simulink model "MPC_temp_arduino"  (R2021a)
settings: Solver=VariableStepAuto  StartTime=0.0  StopTime=10.0  RelTol=1e-3
values from neighbouring files (symbols this model uses):
  A = [0,                              1,                                                           0,                                                            0 ... (first row only)    [ss_mpc.m]    (also in tumbllerDT0.m = [3.9200 -5.7860 3.8100 -0.9451;1 0 0 0;0 1 0 0;0 0 1 0]; tumbller_mpc.m)
  B = v_to_force*[               0 ... (first row only)    [ss_mpc.m]    (also in tumbllerDT0.m = [1;0;0;0]; tumbller_mpc.m = [               0)
  f = 0.01    [ss_mpc.m]    (also in tumbller_mpc.m)
  g = 9.81    [ss_mpc.m]    (also in tumbller_mpc.m)
  I_pend = 0.00024    [ss_mpc.m]    (also in tumbller_mpc.m)
  l = 0.04    [ss_mpc.m]    (also in tumbller_mpc.m)
  m_cart = 0.493    [ss_mpc.m]    (also in tumbller_mpc.m)
  m_pend = 0.312    [ss_mpc.m]    (also in tumbller_mpc.m)
  v_to_force = (2*kT)/(R*r)    (= 0.65671641791)    [ss_mpc.m]    (also in tumbller_mpc.m)
libraries: pid_lib x2, mpclib x1, simulink x1
settings Model: Creator=navoditchandra  LastModifiedBy=navoditchandra

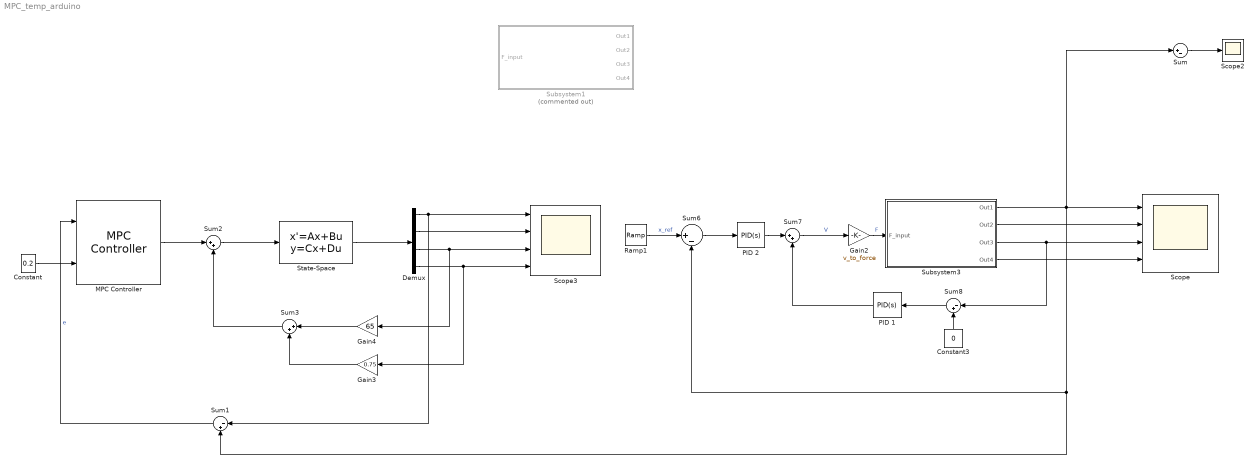
== system MPC_temp_arduino ==
  Constant : Constant  Value=0.2
  Constant3 : Constant  Value=0
  Demux : Demux
  Gain2 : Gain  Gain=v_to_force
  Gain3 : Gain  Gain=0.75
  Gain4 : Gain  Gain=65
  MPC Controller : mpclib/MPC Controller  SCDEnableBlockLinearizationSpecification=on  mpcobj=mpc1  is_multiple=0  enable_value=0  return_u0=off  updateMPCinCallerWorkspace=on  md_inport=off  mv_inport=off  uref_inport=off  return_cost=off  return_mvseq=off  return_qpstatus=off  return_xseq=off  return_state=off  return_ovseq=off  state_inport=off  umin_inport=off  umax_inport=off  ymin_inport=off  ymax_inport=off  cc_inport=off  ywt_inport=off  uwt_inport=off  duwt_inport=off  rhoeps_inport=off  pm_inport=off  MaximumP=10  HorizonChoice=FixedHorizon  n_ts=0.02  n_p=10  n_mv=1  n_md=0  n_ud=0  n_mo=1  n_uo=0  BlockDataType=double  SampleTimeInherited=off  switch_inport=off
  PID 1 : pid_lib/PID Controller  Controller=PID  Form=Parallel  TimeDomain=Continuous-time  UseExternalTs=off  SampleTime=-1  IntegratorMethod=Forward Euler  FilterMethod=Forward Euler  ControllerParametersSource=internal  P=-887.275388547678  I=-21478.8660944054  D=-9.12643726781358  UseFilter=on  N=21022.2428165113  TunerSelectOption=Transfer Function Based (PID Tuner App)  InitialConditionSource=internal  InitialConditionForIntegrator=0  InitialConditionForFilter=0  DifferentiatorICPrevScaledInput=0  ExternalReset=none  TrackingMode=off  Kt=1  LimitOutput=off  SatLimitsSource=internal  UpperSaturationLimit=inf  LowerSaturationLimit=-inf  LinearizeAsGain=on  AntiWindupMode=none  Kb=1  POutMin=[]  POutMax=[]  IOutMin=[]  IOutMax=[]  DOutMin=[]  DOutMax=[]  NOutMin=[]  NOutMax=[]  SumOutMin=[]  SumOutMax=[]  SaturationOutMin=[]  SaturationOutMax=[]  PParamMin=[]  PParamMax=[]  IParamMin=[]  IParamMax=[]  DParamMin=[]  DParamMax=[]  NParamMin=[]  NParamMax=[]  KbParamMin=[]  KbParamMax=[]  KtParamMin=[]  KtParamMax=[]  KbOutMin=[]  KbOutMax=[]  KtOutMin=[]  KtOutMax=[]  IntegratorOutMin=[]  IntegratorOutMax=[]  FilterOutMin=[]  FilterOutMax=[]  SumI1OutMin=[]  SumI1OutMax=[]  SumI2OutMin=[]  SumI2OutMax=[]  SumI3OutMin=[]  SumI3OutMax=[]  SumI4OutMin=[]  SumI4OutMax=[]  SumDOutMin=[]  SumDOutMax=[]  DifferentiatorOutMin=[]  DifferentiatorOutMax=[]  FilterDiffOutCoefMin=[]  FilterDiffOutCoefMax=[]  ReciprocalOutMin=[]  ReciprocalOutMax=[]  SumDenOutMin=[]  SumDenOutMax=[]  SumNumOutMin=[]  SumNumOutMax=[]  DivideOutMin=[]  DivideOutMax=[]  UdiffTsProdOutMin=[]  UdiffTsProdOutMax=[]  NTsProdOutMin=[]  NTsProdOutMax=[]  UintegralTsProdOutMin=[]  UintegralTsProdOutMax=[]  UngainTsProdOutMin=[]  UngainTsProdOutMax=[]  IntegratorContinuousStateAttributes=''  IntegratorStateMustResolveToSignalObject=off  IntegratorRTWStateStorageClass=Auto  FilterContinuousStateAttributes=''  FilterStateMustResolveToSignalObject=off  FilterRTWStateStorageClass=Auto  ParallelPVariant=InternalParameters  IdealPVariant=Disabled  IVariant=InternalParameters  DVariant=InternalParameters  IntegratorVariant=Continuous  SatVariant=Disabled  AWVariant=Passthrough  PCopyVariant=Disabled  TRVariant=Disabled  FdbkBlocksVariant=Forward  IdealPFdbkVariant=Disabled  SatFdbkVariant=Disabled  DerivativeFilterVariant=ContFilter  NVariant=InternalParameters  NCopyVariant=Disabled  FilterICVariant=InternalICsFilter  IntegratorICVariant=InternalICs  ExternalResetVariant=Disabled  TRSumVariant=Passthrough  SumFdbkVariant=Disabled  SumVariant=Sum_PID  TsampFilterVariant=InternalTs  TsampNgainVariant=Passthrough  TsampIntegralVariant=Passthrough  ExternalSaturationOutDataTypeStr=Inherit: Same as second input
  PID 2 : pid_lib/PID Controller  Controller=PID  Form=Parallel  TimeDomain=Continuous-time  UseExternalTs=off  SampleTime=-1  IntegratorMethod=Forward Euler  FilterMethod=Forward Euler  ControllerParametersSource=internal  P=19501.8727650453  I=12310.6101317188  D=-477.528521319051  UseFilter=on  N=35.5633957258041  TunerSelectOption=Transfer Function Based (PID Tuner App)  InitialConditionSource=internal  InitialConditionForIntegrator=0  InitialConditionForFilter=0  DifferentiatorICPrevScaledInput=0  ExternalReset=none  TrackingMode=off  Kt=1  LimitOutput=off  SatLimitsSource=internal  UpperSaturationLimit=inf  LowerSaturationLimit=-inf  LinearizeAsGain=on  AntiWindupMode=none  Kb=1  POutMin=[]  POutMax=[]  IOutMin=[]  IOutMax=[]  DOutMin=[]  DOutMax=[]  NOutMin=[]  NOutMax=[]  SumOutMin=[]  SumOutMax=[]  SaturationOutMin=[]  SaturationOutMax=[]  PParamMin=[]  PParamMax=[]  IParamMin=[]  IParamMax=[]  DParamMin=[]  DParamMax=[]  NParamMin=[]  NParamMax=[]  KbParamMin=[]  KbParamMax=[]  KtParamMin=[]  KtParamMax=[]  KbOutMin=[]  KbOutMax=[]  KtOutMin=[]  KtOutMax=[]  IntegratorOutMin=[]  IntegratorOutMax=[]  FilterOutMin=[]  FilterOutMax=[]  SumI1OutMin=[]  SumI1OutMax=[]  SumI2OutMin=[]  SumI2OutMax=[]  SumI3OutMin=[]  SumI3OutMax=[]  SumI4OutMin=[]  SumI4OutMax=[]  SumDOutMin=[]  SumDOutMax=[]  DifferentiatorOutMin=[]  DifferentiatorOutMax=[]  FilterDiffOutCoefMin=[]  FilterDiffOutCoefMax=[]  ReciprocalOutMin=[]  ReciprocalOutMax=[]  SumDenOutMin=[]  SumDenOutMax=[]  SumNumOutMin=[]  SumNumOutMax=[]  DivideOutMin=[]  DivideOutMax=[]  UdiffTsProdOutMin=[]  UdiffTsProdOutMax=[]  NTsProdOutMin=[]  NTsProdOutMax=[]  UintegralTsProdOutMin=[]  UintegralTsProdOutMax=[]  UngainTsProdOutMin=[]  UngainTsProdOutMax=[]  IntegratorContinuousStateAttributes=''  IntegratorStateMustResolveToSignalObject=off  IntegratorRTWStateStorageClass=Auto  FilterContinuousStateAttributes=''  FilterStateMustResolveToSignalObject=off  FilterRTWStateStorageClass=Auto  ParallelPVariant=InternalParameters  IdealPVariant=Disabled  IVariant=InternalParameters  DVariant=InternalParameters  IntegratorVariant=Continuous  SatVariant=Disabled  AWVariant=Passthrough  PCopyVariant=Disabled  TRVariant=Disabled  FdbkBlocksVariant=Forward  IdealPFdbkVariant=Disabled  SatFdbkVariant=Disabled  DerivativeFilterVariant=ContFilter  NVariant=InternalParameters  NCopyVariant=Disabled  FilterICVariant=InternalICsFilter  IntegratorICVariant=InternalICs  ExternalResetVariant=Disabled  TRSumVariant=Passthrough  SumFdbkVariant=Disabled  SumVariant=Sum_PID  TsampFilterVariant=InternalTs  TsampNgainVariant=Passthrough  TsampIntegralVariant=Passthrough  ExternalSaturationOutDataTypeStr=Inherit: Same as second input
  Ramp1 : simulink/Sources/Ramp  slope=1  start=0  InitialOutput=0
  Scope : Scope  NumInputPorts=4
  Scope2 : Scope
  Scope3 : Scope  NumInputPorts=4
  State-Space : StateSpace  A=A  B=B  C=eye(4)  D=zeros(4,1)  InitialCondition=-0.2
  Subsystem1 : Subsystem  Commented=on
  Subsystem3 : Subsystem
  Sum : Sum  Inputs=|+-
  Sum1 : Sum  Inputs=|-+
  Sum2 : Sum  Inputs=|++
  Sum3 : Sum  Inputs=|++
  Sum6 : Sum  Inputs=|+-
  Sum7 : Sum  Inputs=|++
  Sum8 : Sum  Inputs=|-+
  wires:
  Sum6/1 -> PID 2/1
  PID 1/1 -> Sum7/2
  Subsystem3/1(Out1) -> Sum/1, Sum1/2, Sum6/2, Scope/1
  Sum/1 -> Scope2/1
  MPC Controller/1 -> Sum2/1
  Sum7/1 -> Gain2/1  "V"
  Sum8/1 -> PID 1/1
  Sum2/1 -> State-Space/1
  Sum1/1 -> MPC Controller/1  "e"
  Constant/1 -> MPC Controller/2
  Subsystem3/2(Out2) -> Scope/2
  Gain2/1 -> Subsystem3/1(F_input)  "F"
  Subsystem3/4(Out4) -> Scope/4
  PID 2/1 -> Sum7/1
  Subsystem3/3(Out3) -> Sum8/1, Scope/3
  Ramp1/1 -> Sum6/1  "x_ref"
  Constant3/1 -> Sum8/2
  Gain4/1 -> Sum3/1
  Gain3/1 -> Sum3/2
  Sum3/1 -> Sum2/2
  State-Space/1 -> Demux/1
  Demux/3 -> Scope3/3, Gain4/1
  Demux/4 -> Scope3/4, Gain3/1
  Demux/1 -> Sum1/1, Scope3/1
  Demux/2 -> Scope3/2

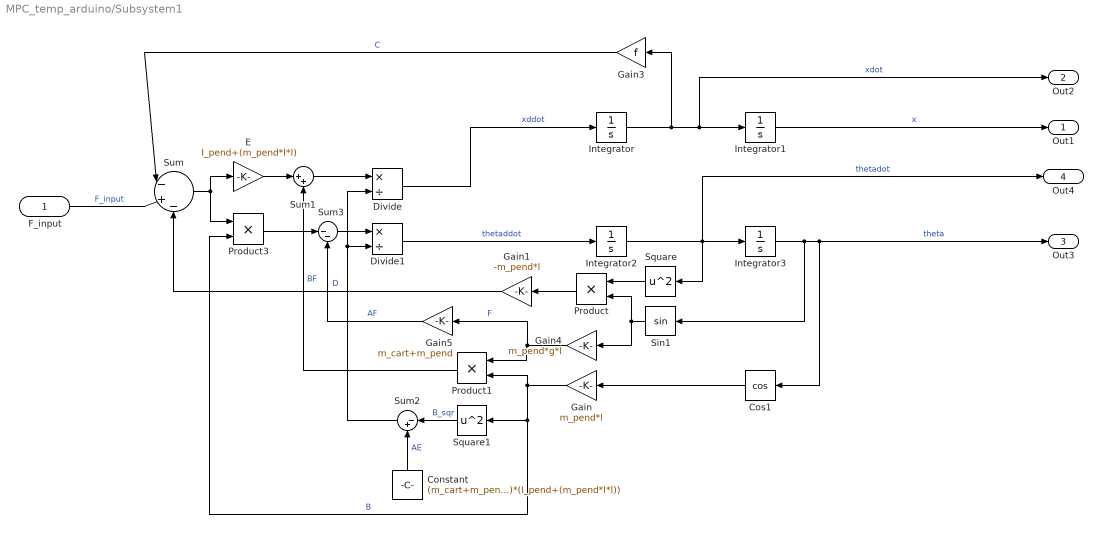
== system MPC_temp_arduino/Subsystem1 ==
  F_input : Inport
  Constant : Constant  Value=(m_cart+m_pend)*(I_pend+(m_pend*l*l))
  Cos1 : Trigonometry  Operator=cos
  Divide : Product  Inputs=*/
  Divide1 : Product  Inputs=*/
  E : Gain  Gain=I_pend+(m_pend*l*l)
  Gain : Gain  Gain=m_pend*l
  Gain1 : Gain  Gain=-m_pend*l
  Gain3 : Gain  Gain=f
  Gain4 : Gain  Gain=m_pend*g*l
  Gain5 : Gain  Gain=m_cart+m_pend
  Integrator : Integrator
  Integrator1 : Integrator  InitialCondition=-0.2
  Integrator2 : Integrator
  Integrator3 : Integrator
  Product : Product
  Product1 : Product
  Product3 : Product
  Sin1 : Trigonometry
  Square : Math  Operator=square  SaturateOnIntegerOverflow=on
  Square1 : Math  Operator=square  SaturateOnIntegerOverflow=on
  Sum : Sum  Inputs=|-+-
  Sum1 : Sum  Inputs=|++
  Sum2 : Sum  Inputs=|-+
  Sum3 : Sum  Inputs=|--
  Out1 : Outport
  Out2 : Outport  Port=2
  Out3 : Outport  Port=3
  Out4 : Outport  Port=4
  wires:
  Integrator2/1 -> Out4/1, Integrator3/1, Square/1  "thetadot"
  Integrator/1 -> Gain3/1, Integrator1/1, Out2/1  "xdot"
  Divide/1 -> Integrator/1  "xddot"
  Divide1/1 -> Integrator2/1  "thetaddot"
  Integrator1/1 -> Out1/1  "x"
  Gain/1 -> Product1/2, Product3/2, Square1/1  "B"
  Cos1/1 -> Gain/1
  Integrator3/1 -> Out3/1, Cos1/1, Sin1/1  "theta"
  Gain3/1 -> Sum/1  "C"
  Sin1/1 -> Gain4/1, Product/2
  Square/1 -> Product/1
  Product/1 -> Gain1/1
  Gain1/1 -> Sum/3  "D"
  Gain4/1 -> Gain5/1, Product1/1  "F"
  F_input/1 -> Sum/2  "F_input"
  Sum/1 -> Product3/1, E/1
  E/1 -> Sum1/1
  Product1/1 -> Sum1/2  "BF"
  Sum1/1 -> Divide/1
  Square1/1 -> Sum2/1  "B_sqr"
  Constant/1 -> Sum2/2  "AE"
  Sum2/1 -> Divide/2, Divide1/2
  Product3/1 -> Sum3/1
  Gain5/1 -> Sum3/2  "AF"
  Sum3/1 -> Divide1/1

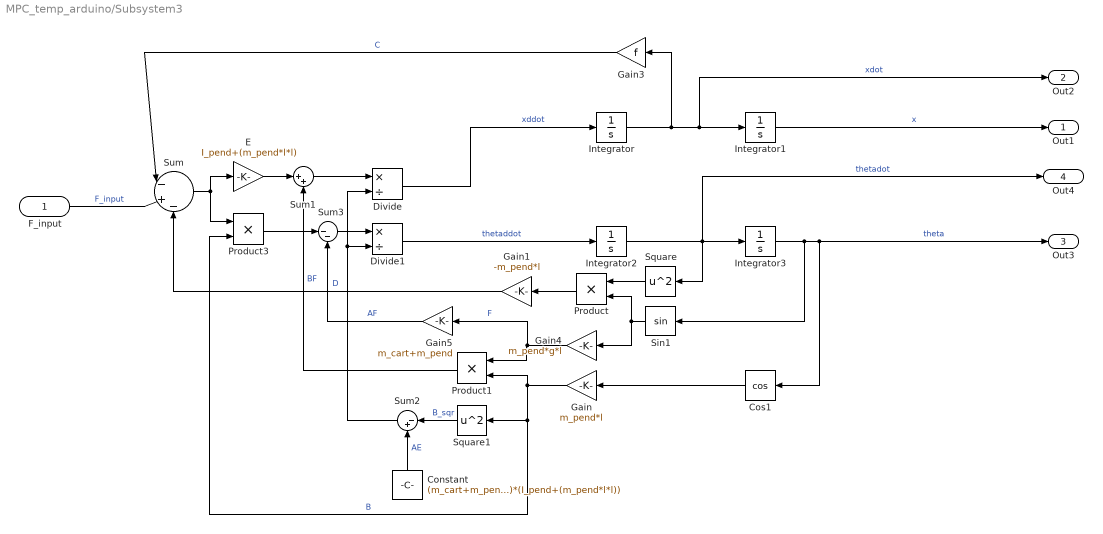
== system MPC_temp_arduino/Subsystem3 ==
  F_input : Inport
  Constant : Constant  Value=(m_cart+m_pend)*(I_pend+(m_pend*l*l))
  Cos1 : Trigonometry  Operator=cos
  Divide : Product  Inputs=*/
  Divide1 : Product  Inputs=*/
  E : Gain  Gain=I_pend+(m_pend*l*l)
  Gain : Gain  Gain=m_pend*l
  Gain1 : Gain  Gain=-m_pend*l
  Gain3 : Gain  Gain=f
  Gain4 : Gain  Gain=m_pend*g*l
  Gain5 : Gain  Gain=m_cart+m_pend
  Integrator{,1..3} (4 alike) : Integrator
  Product : Product
  Product1 : Product
  Product3 : Product
  Sin1 : Trigonometry
  Square : Math  Operator=square  SaturateOnIntegerOverflow=on
  Square1 : Math  Operator=square  SaturateOnIntegerOverflow=on
  Sum : Sum  Inputs=|-+-
  Sum1 : Sum  Inputs=|++
  Sum2 : Sum  Inputs=|-+
  Sum3 : Sum  Inputs=|--
  Out1 : Outport
  Out2 : Outport  Port=2
  Out3 : Outport  Port=3
  Out4 : Outport  Port=4
  wires:
  Integrator2/1 -> Out4/1, Integrator3/1, Square/1  "thetadot"
  Integrator/1 -> Gain3/1, Integrator1/1, Out2/1  "xdot"
  Divide/1 -> Integrator/1  "xddot"
  Divide1/1 -> Integrator2/1  "thetaddot"
  Integrator1/1 -> Out1/1  "x"
  Gain/1 -> Product1/2, Product3/2, Square1/1  "B"
  Cos1/1 -> Gain/1
  Integrator3/1 -> Out3/1, Cos1/1, Sin1/1  "theta"
  Gain3/1 -> Sum/1  "C"
  Sin1/1 -> Gain4/1, Product/2
  Square/1 -> Product/1
  Product/1 -> Gain1/1
  Gain1/1 -> Sum/3  "D"
  Gain4/1 -> Gain5/1, Product1/1  "F"
  F_input/1 -> Sum/2  "F_input"
  Sum/1 -> Product3/1, E/1
  E/1 -> Sum1/1
  Product1/1 -> Sum1/2  "BF"
  Sum1/1 -> Divide/1
  Square1/1 -> Sum2/1  "B_sqr"
  Constant/1 -> Sum2/2  "AE"
  Sum2/1 -> Divide/2, Divide1/2
  Product3/1 -> Sum3/1
  Gain5/1 -> Sum3/2  "AF"
  Sum3/1 -> Divide1/1
